simulink library "lib_iir_filter"  (R2023a)
settings: Solver=VariableStepAuto  StartTime=0.0  StopTime=10.0  RelTol=1e-3
libraries: lib_conversion x5
settings Model: Creator=cav2ofo  LastModifiedBy=lenovo
settings OptimizationCC: ReuseModelBlockBuffer=off

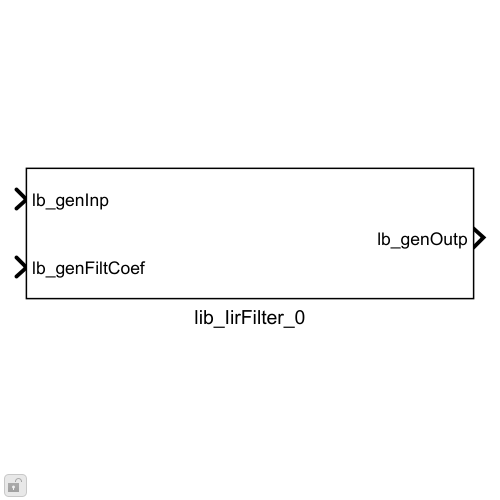
[thumbnail: Simulink's stored preview of the top-level diagram]
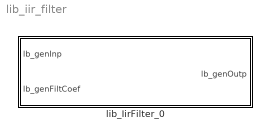
== system lib_iir_filter ==
  lib_IirFilter_0 : Subsystem  mask{lb_parMaxInpVal=1000, lb_parFltrCoefMaxVal=0.02, lb_parBitNumMode=16-bit, lb_parOutpDataType=Inherit: Inherit via back propagation, lb_parFiltTypeMode=Low-pass}
      mask prompts: lb_parMaxInpVal "Input signal max value:"; lb_parFltrCoefMaxVal "Filter coefficient max value:"; lb_parBitNumMode "Bits number for internal calculations:"; lb_parOutpDataType "Output data type:"; lb_parFiltTypeMode "Filter type:"
      mask init:
      | % %Re-initialize parameters in Double
      | % lb_parMaxInpVal = double(lb_parMaxInpVal);
      | % lb_parFltrCoefMaxVal = double(lb_parFltrCoefMaxVal);
      | % 
      | % % Data type for the derivative of the input signal
      | % lb_parInpDrvtMaxVal = lb_parMaxInpVal*lb_parFltrCoefMaxVal;
      | % lb_parInpDrvtDataType = Simulink.NumericType;
      | % lb_parInpDrvtDataType.Signedness = 'Signed';
      | % lb_parInpDrvtDataType.DataTypeMode= 'Fixed-point: unspecified scaling';
      | % if lb_parInpDrvtMaxVal <= (2^15)-1
      | %     lb_parInpDrvtDataType.WordLength = 16;
      | % else
      | %     lb_parInpDrvtDataType.WordLength = 32;
      | % end
      | 
      | switch lb_parFiltTypeMode
      |     case 'Low-pass'
      |         set_param([gcb,'/vss_FilterVariant'],'LabelModeActiveChoice','lb_parLowPassModeLbl');
      |     case 'High-pass'
      |         set_param([gcb,'/vss_FilterVariant'],'LabelModeActiveChoice','lb_parHighPassModeLbl');
      | end
      | 
      | switch lb_parBitNumMode
      |     case '16-bit'
      |         lb_parBitNum = 16;
      |     case '32-bit'
      |         lb_parBitNum = 32;
      |     otherwise
      |         lb_parBitNum = 16;
      | end
      mask TypeOptions lb_parBitNumMode: 16-bit | 32-bit
      mask TypeOptions lb_parFiltTypeMode: Low-pass | High-pass
      mask DialogControl DescGroupVar Prompt: VHIT IIR filter
      mask DialogControl DescTextVar Prompt: This block implements implements a discrete-time first order low-pass IIR filter
      mask DialogControl dataTypeDesc Prompt: Data type
      mask DialogControl dataTypeDesc_copy Prompt: Operating mode

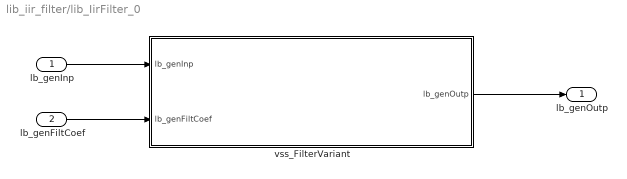
== system lib_iir_filter/lib_IirFilter_0 ==
  lb_genInp : Inport
  lb_genFiltCoef : Inport  Port=2
  vss_FilterVariant : Subsystem  Variant=on  VariantControlMode=label  LabelModeActiveChoice=lb_parLowPassModeLbl
  lb_genOutp : Outport  VectorParamsAs1DForOutWhenUnconnected=off
  wires:
  lb_genInp/1 -> vss_FilterVariant/1(lb_genInp)
  lb_genFiltCoef/1 -> vss_FilterVariant/2(lb_genFiltCoef)
  vss_FilterVariant/1(lb_genOutp) -> lb_genOutp/1

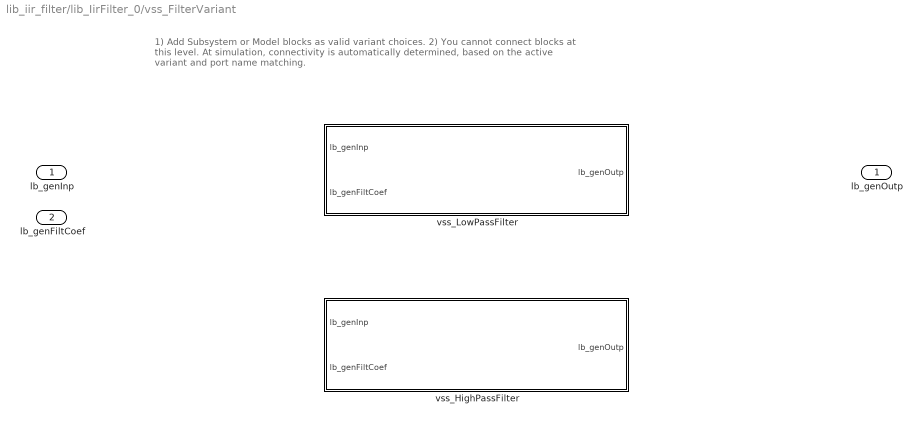
== system lib_iir_filter/lib_IirFilter_0/vss_FilterVariant ==
  note: 1) Add Subsystem or Model blocks as valid variant choices.
      | 2) You cannot connect blocks at this level. At simulation, connectivity is automatically
      | determined, based on the active variant and port name matching.
  lb_genInp : Inport
  lb_genFiltCoef : Inport  Port=2
  vss_HighPassFilter : Subsystem  VariantControl=lb_parHighPassModeLbl
  vss_LowPassFilter : Subsystem  VariantControl=lb_parLowPassModeLbl
  lb_genOutp : Outport

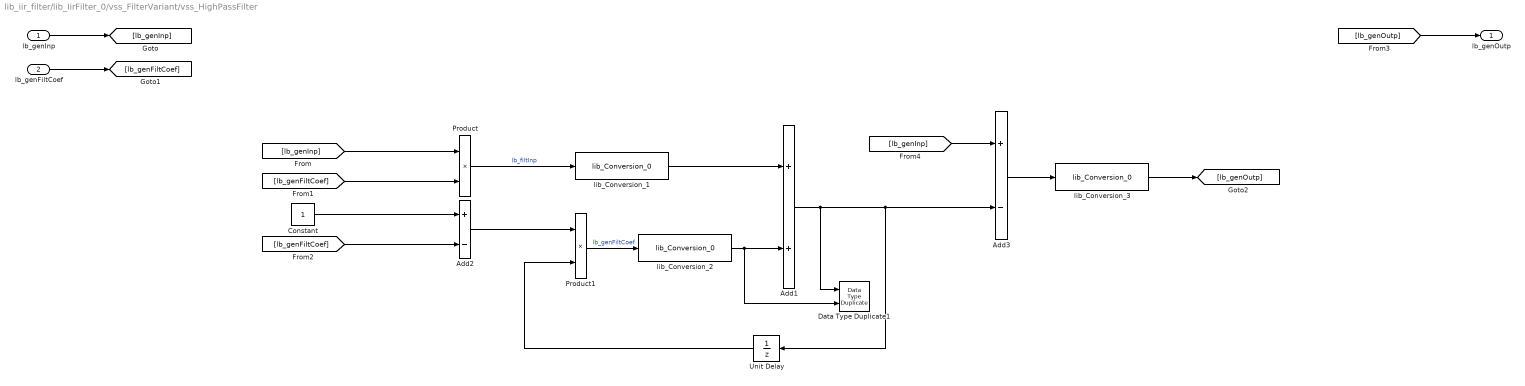
== system lib_iir_filter/lib_IirFilter_0/vss_FilterVariant/vss_HighPassFilter ==
  lb_genInp : Inport
  lb_genFiltCoef : Inport  Port=2
  Add1 : Sum  OutDataTypeStr=Inherit: Inherit via back propagation  RndMeth=Simplest
  Add2 : Sum  Inputs=+-  RndMeth=Simplest  OutDataTypeStr=Inherit: Same as first input
  Add3 : Sum  Inputs=+-  OutDataTypeStr=Inherit: Inherit via back propagation  RndMeth=Simplest
  Constant : Constant  OutDataTypeStr=fixdt(0,16,2^-15,0)
  Data Type Duplicate1 : DataTypeDuplicate
  Product : Product  OutDataTypeStr=Inherit: Inherit via back propagation  RndMeth=Simplest
  Product1 : Product  OutDataTypeStr=Inherit: Inherit via back propagation  RndMeth=Simplest
  Unit Delay : UnitDelay  SampleTime=-1  HasFrameUpgradeWarning=on
  lib_Conversion_1 : lib_conversion/lib_Conversion_0  lb_parDataType=fixdt(1,lb_parBitNum)  lb_parOutpMaxVal=lb_parMaxInpVal*lb_parFltrCoefMaxVal  lb_parOutpMinVal=[]  lb_parSatFlag=off
  lib_Conversion_2 : lib_conversion/lib_Conversion_0  lb_parDataType=fixdt(1,lb_parBitNum)  lb_parOutpMaxVal=lb_parMaxInpVal  lb_parOutpMinVal=[]  lb_parSatFlag=off
  lib_Conversion_3 : lib_conversion/lib_Conversion_0  lb_parDataType=lb_parOutpDataType  lb_parOutpMaxVal=[]  lb_parOutpMinVal=[]  lb_parSatFlag=off
  lb_genOutp : Outport  VectorParamsAs1DForOutWhenUnconnected=off
  wires:
  Add1/1 -> Data Type Duplicate1/1, Unit Delay/1, Add3/2
  Add2/1 -> Product1/1
  [lb_genInp] -> Product/1
  lib_Conversion_1/1 -> Add1/1
  Unit Delay/1 -> Product1/2
  lib_Conversion_2/1 -> Add1/2, Data Type Duplicate1/2
  [lb_genFiltCoef] -> Add2/2
  Product1/1 -> lib_Conversion_2/1  "lb_genFiltCoef"
  lb_genInp/1 -> [lb_genInp]
  Constant/1 -> Add2/1
  [lb_genFiltCoef] -> Product/2
  [lb_genOutp] -> lb_genOutp/1
  lb_genFiltCoef/1 -> [lb_genFiltCoef]
  lib_Conversion_3/1 -> [lb_genOutp]
  Product/1 -> lib_Conversion_1/1  "lb_filtInp"
  [lb_genInp] -> Add3/1
  Add3/1 -> lib_Conversion_3/1

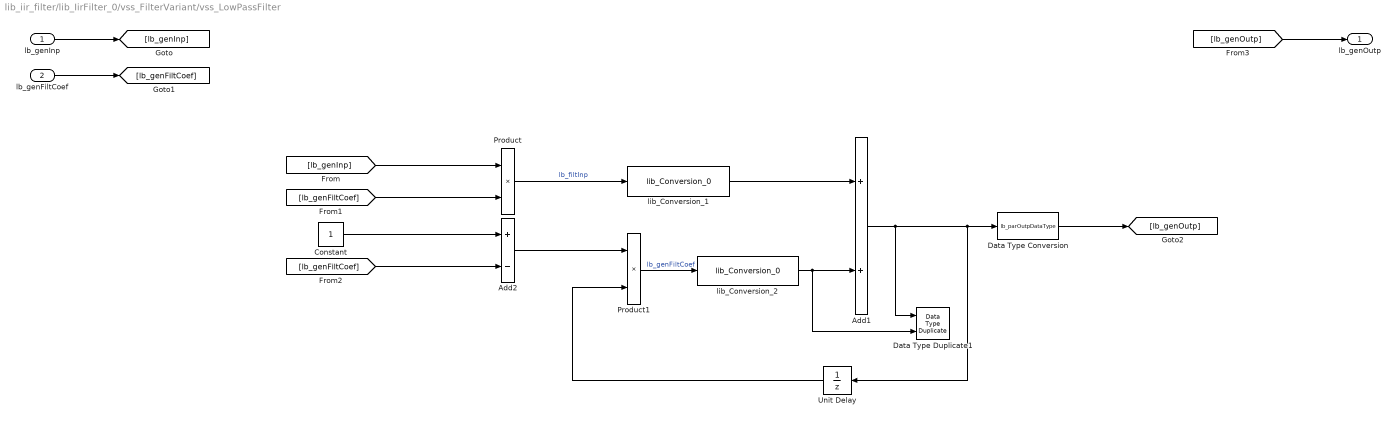
== system lib_iir_filter/lib_IirFilter_0/vss_FilterVariant/vss_LowPassFilter ==
  lb_genInp : Inport
  lb_genFiltCoef : Inport  Port=2
  Add1 : Sum  OutDataTypeStr=Inherit: Inherit via back propagation  RndMeth=Simplest
  Add2 : Sum  Inputs=+-  RndMeth=Simplest  OutDataTypeStr=Inherit: Same as first input
  Constant : Constant  OutDataTypeStr=fixdt(0,16,2^-15,0)
  Data Type Duplicate1 : DataTypeDuplicate
  Data Type Conversion : DataTypeConversion  OutDataTypeStr=lb_parOutpDataType  SaturateOnIntegerOverflow=off  RndMeth=Floor
  Product : Product  OutDataTypeStr=Inherit: Inherit via back propagation  RndMeth=Simplest
  Product1 : Product  OutDataTypeStr=Inherit: Inherit via back propagation  RndMeth=Simplest
  Unit Delay : UnitDelay  SampleTime=-1  HasFrameUpgradeWarning=on
  lib_Conversion_1 : lib_conversion/lib_Conversion_0  lb_parDataType=fixdt(1,lb_parBitNum)  lb_parOutpMaxVal=lb_parMaxInpVal*lb_parFltrCoefMaxVal  lb_parOutpMinVal=[]  lb_parSatFlag=off
  lib_Conversion_2 : lib_conversion/lib_Conversion_0  lb_parDataType=fixdt(1,lb_parBitNum)  lb_parOutpMaxVal=lb_parMaxInpVal  lb_parOutpMinVal=[]  lb_parSatFlag=off
  lb_genOutp : Outport  VectorParamsAs1DForOutWhenUnconnected=off
  wires:
  lb_genInp/1 -> [lb_genInp]
  Add1/1 -> Data Type Duplicate1/1, Data Type Conversion/1, Unit Delay/1
  Add2/1 -> Product1/1
  Product/1 -> lib_Conversion_1/1  "lb_filtInp"
  lb_genFiltCoef/1 -> [lb_genFiltCoef]
  Product1/1 -> lib_Conversion_2/1  "lb_genFiltCoef"
  lib_Conversion_1/1 -> Add1/1
  [lb_genFiltCoef] -> Add2/2
  Constant/1 -> Add2/1
  [lb_genFiltCoef] -> Product/2
  [lb_genInp] -> Product/1
  Unit Delay/1 -> Product1/2
  lib_Conversion_2/1 -> Add1/2, Data Type Duplicate1/2
  Data Type Conversion/1 -> [lb_genOutp]
  [lb_genOutp] -> lb_genOutp/1
